simulink model "sim_Ex1"  (R2022b)
settings: Solver=VariableStepAuto  StartTime=0.0  StopTime=10.0  RelTol=1e-3
settings Model: Creator=MAAM  LastModifiedBy=MAAM

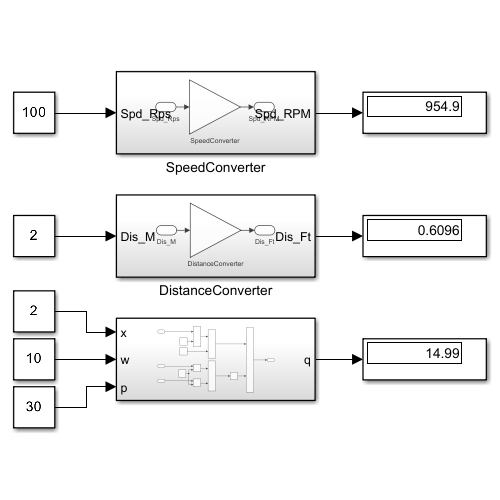
[thumbnail: Simulink's stored preview of the top-level diagram]
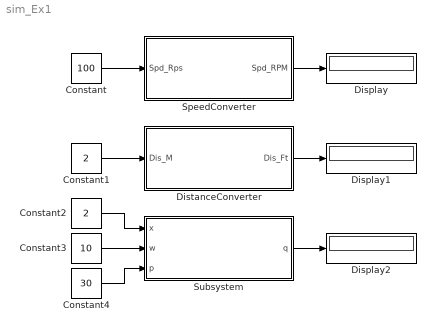
== system sim_Ex1 ==
  Constant : Constant  Value=100
  Constant1 : Constant  Value=2
  Constant2 : Constant  Value=2
  Constant3 : Constant  Value=10
  Constant4 : Constant  Value=30
  Display : Display
  Display1 : Display
  Display2 : Display
  DistanceConverter : Subsystem
  SpeedConverter : Subsystem
  Subsystem : Subsystem
  wires:
  Constant/1 -> SpeedConverter/1(Spd_Rps)
  SpeedConverter/1(Spd_RPM) -> Display/1
  Constant1/1 -> DistanceConverter/1(Dis_M)
  DistanceConverter/1(Dis_Ft) -> Display1/1
  Constant3/1 -> Subsystem/2(w)
  Constant2/1 -> Subsystem/1(x)
  Constant4/1 -> Subsystem/3(p)
  Subsystem/1(q) -> Display2/1

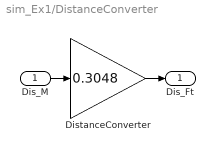
== system sim_Ex1/DistanceConverter ==
  Dis_M : Inport
  DistanceConverter : Gain  Gain=0.3048
  Dis_Ft : Outport
  wires:
  Dis_M/1 -> DistanceConverter/1
  DistanceConverter/1 -> Dis_Ft/1

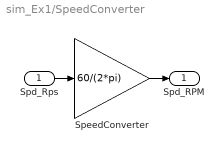
== system sim_Ex1/SpeedConverter ==
  Spd_Rps : Inport
  SpeedConverter : Gain  Gain=60/(2*pi)
  Spd_RPM : Outport
  wires:
  SpeedConverter/1 -> Spd_RPM/1
  Spd_Rps/1 -> SpeedConverter/1

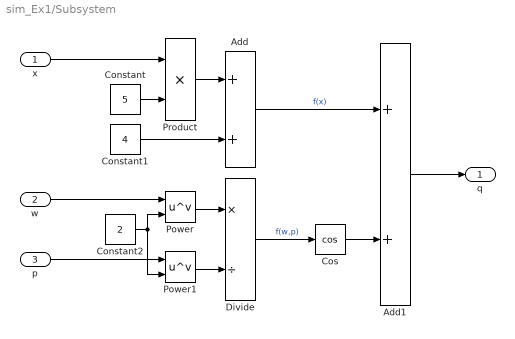
== system sim_Ex1/Subsystem ==
  x : Inport
  w : Inport  Port=2
  p : Inport  Port=3
  Add : Sum
  Add1 : Sum
  Constant : Constant  Value=5
  Constant1 : Constant  Value=4
  Constant2 : Constant  Value=2
  Cos : Trigonometry  Operator=cos
  Divide : Product  Inputs=*/
  Power : Math  Operator=pow
  Power1 : Math  Operator=pow
  Product : Product
  q : Outport
  wires:
  x/1 -> Product/1
  Product/1 -> Add/1
  Constant/1 -> Product/2
  Constant1/1 -> Add/2
  Add/1 -> Add1/1  "f(x)"
  w/1 -> Power/1
  Constant2/1 -> Power1/2, Power/2
  p/1 -> Power1/1
  Power/1 -> Divide/1
  Power1/1 -> Divide/2
  Divide/1 -> Cos/1  "f(w,p)"
  Cos/1 -> Add1/2
  Add1/1 -> q/1
